simulink model "model2"  (R2024b)
settings: Solver=VariableStepAuto  StartTime=0.0  StopTime=10.0  MaxStep=5  RelTol=1e-3
values from neighbouring files (symbols this model uses):
  A = [ -Kg/cvg,     Kg/cvg ... (first row only)    [Lab1cz2.m]
  B = [ 1/cvg,        0 ... (first row only)    [Lab1cz2.m]
  C = [ 1, 0 ... (first row only)    [Lab1cz2.m]
  D = [ 0, 0 ... (first row only)    [Lab1cz2.m]
  dPg = 0    [Lab1.m]    (also in Lab1cz2.m)
  dTzew = 1    [Lab1.m]    (also in Lab1cz2.m)
  Pg0 = tab_Pg(i)    [Lab1.m]    (also in Lab1cz2.m)
  Tg0 = (Pg0+Kg*Twew0)/Kg    [Lab1.m]    (also in Lab1cz2.m = x(1))
  Twew0 = (Pg0+(K1+K2)*Tzew0)/(K1+K2)    [Lab1.m]    (also in Lab1cz2.m = x(2))
  Tzew0 = tab_Tzew(i)    [Lab1.m]    (also in Lab1cz2.m)
settings Model: Creator=konra  LastModifiedBy=konra

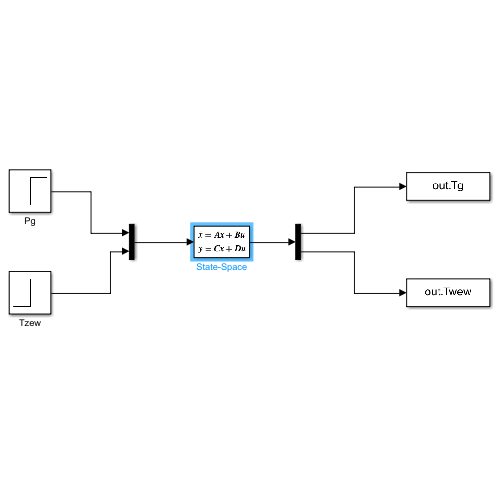
[thumbnail: Simulink's stored preview of the top-level diagram]
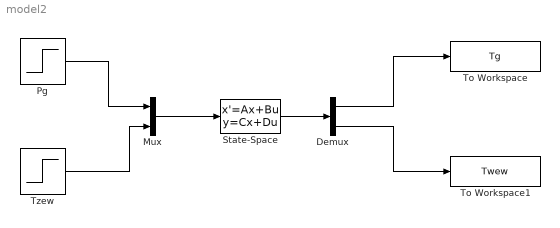
== system model2 ==
  Demux : Demux  Outputs=2
  Mux : Mux  Inputs=2
  Pg : Step  Time=5000  Before=Pg0  After=Pg0+dPg  SampleTime=0
  State-Space : StateSpace  A=A  B=B  C=C  D=D  InitialCondition=[Tg0, Twew0]  AllowTunableDMatrix=on
  To Workspace : ToWorkspace  VariableName=Tg  SampleTime=-1
  To Workspace1 : ToWorkspace  VariableName=Twew  SampleTime=-1
  Tzew : Step  Time=5000  Before=Tzew0  After=Tzew0+dTzew  SampleTime=0
  wires:
  Pg/1 -> Mux/1
  Tzew/1 -> Mux/2
  Mux/1 -> State-Space/1
  State-Space/1 -> Demux/1
  Demux/1 -> To Workspace/1
  Demux/2 -> To Workspace1/1
